simulink model "Combined_Experiment_Mar25_2020a_TorqueControl"  (R2020a)
settings: Solver=FixedStepAuto  StartTime=0.0  StopTime=tsim  FixedStep=baseRate  MaxStep=0.0001  RelTol=1e-6  AbsTol=1e-6  EnableMultiTasking=on
values from neighbouring files (symbols this model uses):
  b0 = importdata("biases_layer_0.csv")    [Run_Initializer.m]
  b1 = importdata("biases_layer_1.csv")    [Run_Initializer.m]
  b_out = importdata("biases_output.csv")    [Run_Initializer.m]
  baseRate = 0.05    [Run_Initializer.m]
  CHASER_ABSOLUTE_POSITION = true    [Run_Initializer.m]
  drop_states_ARM = [ pi/2, pi/2, 0]    [Run_Initializer.m]
  drop_states_BLACK = [ xLength/2, yLength/2, pi]    [Run_Initializer.m]
  drop_states_BLUE = [ xLength/2, yLength/2, pi]    [Run_Initializer.m]
  drop_states_RED = [ xLength/2+0.5, yLength/2, pi]    [Run_Initializer.m]
  F_Black_X_nominal = 0.2196    [Run_Initializer.m]
  F_Black_Y_nominal = 0.2825    [Run_Initializer.m]
  F_Blue_X_nominal = 0.2196    [Run_Initializer.m]
  F_Blue_Y_nominal = 0.2825    [Run_Initializer.m]
  F_red_X_nominal = 0.2196    [Run_Initializer.m]
  F_red_Y_nominal = 0.2825    [Run_Initializer.m]
  F_thrusters_BLACK = [F_Black_X_nominal; F_Black_X_nominal;                             F_Black_Y_nominal; F_Black_Y_nominal; F_Black_X_nominal;                              F_Black_X_nominal; F_Black_Y_nominal; F_Black_Y_nominal]    [Run_Initializer.m]
  F_thrusters_BLUE = [F_Blue_X_nominal; F_Blue_X_nominal;                             F_Blue_Y_nominal; F_Blue_Y_nominal; F_Blue_X_nominal;                              F_Blue_X_nominal; F_Blue_Y_nominal; F_Blue_Y_nominal]    [Run_Initializer.m]
  F_thrusters_RED = [F_red_X_nominal; F_red_X_nominal;                             F_red_Y_nominal; F_red_Y_nominal; F_red_X_nominal;                              F_red_X_nominal; F_red_Y_nominal; F_red_Y_nominal]    [Run_Initializer.m]
  Gamma1_el = 0.12    [Run_Initializer.m]
  Gamma1_sh = 0.005    [Run_Initializer.m]
  Gamma1_wr = 0.025    [Run_Initializer.m]
  Gamma2_el = 5    [Run_Initializer.m]
  Gamma2_sh = 15    [Run_Initializer.m]
  Gamma2_wr = 5    [Run_Initializer.m]
  Gamma3_el = 10    [Run_Initializer.m]
  Gamma3_sh = 40    [Run_Initializer.m]
  Gamma3_wr = 40    [Run_Initializer.m]
  Gamma4_el = 0.039    [Run_Initializer.m]
  Gamma4_sh = 0.015    [Run_Initializer.m]
  Gamma4_wr = 0.029    [Run_Initializer.m]
  Gamma5_el = 800    [Run_Initializer.m]
  Gamma5_sh = 800    [Run_Initializer.m]
  Gamma5_wr = 800    [Run_Initializer.m]
  Gamma6_el = 0.000001    (= 1e-06)    [Run_Initializer.m]
  Gamma6_sh = 0.005    [Run_Initializer.m]
  Gamma6_wr = 0.02    [Run_Initializer.m]
  HOLD_POINT_RADIUS = 0.95    [Run_Initializer.m]
  home_states_BLACK = [ xLength/2; yLength/2; 0]    [Run_Initializer.m]
  home_states_BLUE = [ xLength/2; yLength/2; 0]    [Run_Initializer.m]
  home_states_RED = [ xLength/2+0.9; yLength/2; pi]    [Run_Initializer.m]
  init_states_BLACK = [ xLength/2; yLength/2; pi]    [Run_Initializer.m]
  init_states_BLUE = [ xLength/2; yLength/2; pi]    [Run_Initializer.m]
  init_states_RED = [ xLength/2+0.9; yLength/2; pi]    [Run_Initializer.m]
  Kd_tb = 1.0    (= 1)    [Run_Initializer.m]
  Kd_tblue = 1    [Run_Initializer.m]
  Kd_tr = 1.0    (= 1)    [Run_Initializer.m]
  Kd_xb = 8    [Run_Initializer.m]
  Kd_xblue = 8    [Run_Initializer.m]
  Kd_xr = 8    [Run_Initializer.m]
  Kd_yb = 8    [Run_Initializer.m]
  Kd_yblue = 8    [Run_Initializer.m]
  Kd_yr = 8    [Run_Initializer.m]
  Kp_tb = 0.1    [Run_Initializer.m]
  Kp_tblue = 0.1    [Run_Initializer.m]
  Kp_tr = 0.1    [Run_Initializer.m]
  Kp_xb = 2    [Run_Initializer.m]
  Kp_xblue = 2    [Run_Initializer.m]
  Kp_xr = 2    [Run_Initializer.m]
  Kp_yb = 2    [Run_Initializer.m]
  Kp_yblue = 2    [Run_Initializer.m]
  Kp_yr = 2    [Run_Initializer.m]
  MAX_BODY_ANGULAR_VELOCITY = 15*180/pi    (= 859.436692696)    [Run_Initializer.m]
  MAX_VELOCITY = 0.1    [Run_Initializer.m]
  noise_variance_BLACK = 0    [Run_Initializer.m]
  noise_variance_BLUE = 0    [Run_Initializer.m]
  noise_variance_RED = 0    [Run_Initializer.m]
  Phase0_End = Phase0_Duration    (= 10)    [Run_Initializer.m]
  Phase1_End = Phase0_Duration + Phase1_Duration    (= 15)    [Run_Initializer.m]
  Phase2_End = Phase0_Duration + Phase1_Duration +                                   Phase2_Duration    (= 45)    [Run_Initializer.m]
  Phase3_End = Phase0_Duration + Phase1_Duration +                                   Phase2_Duration + Phase3_Duration    (= 560)    [Run_Initializer.m]
  Phase3_SubPhase1_End = Phase2_End + Phase3_SubPhase1_Duration    (= 105)    [Run_Initializer.m]
  Phase3_SubPhase2_End = Phase2_End + Phase3_SubPhase1_Duration +                                   Phase3_SubPhase2_Duration    (= 210)    [Run_Initializer.m]
  Phase3_SubPhase3_End = Phase2_End + Phase3_SubPhase1_Duration +                                   Phase3_SubPhase2_Duration +                                  Phase3_SubPhase3_Duration    (= 240)    [Run_Initializer.m]
  Phase3_SubPhase4_End = Phase2_End + Phase3_SubPhase1_Duration +                                   Phase3_SubPhase2_Duration +                                  Phase3_SubPhase3_Duration +                                  Phase3_SubPhase4_Duration    [Run_Initializer.m]
  Phase4_End = Phase0_Duration + Phase1_Duration +                                   Phase2_Duration + Phase3_Duration +                                   Phase4_Duration    (= 680)    [Run_Initializer.m]
  Phase5_End = Phase0_Duration + Phase1_Duration +                                   Phase2_Duration + Phase3_Duration +                                   Phase4_Duration + Phase5_Duration    (= 700)    [Run_Initializer.m]
  relevant_half_range = (upper_state_bound - lower_state_bound)/2    [Run_Initializer.m]
  relevant_state_mean = (lower_state_bound + upper_state_bound)/2    [Run_Initializer.m]
  thruster_dist2CG_BLACK = [72.80;-65.20;61.75;-79.75;65.20;-65.20;74.25;-54.75]    [Run_Initializer.m]
  thruster_dist2CG_BLUE = [83.10;-54.90;71.50;-70.00;54.90;-75.50;64.50;-64.50]    [Run_Initializer.m]
  thruster_dist2CG_RED = [69.38;-56.62;50.01;-81.49;61.12;-68.38;78.99;-52.01]    [Run_Initializer.m]
  w0 = importdata("weights_layer_0.csv")    [Run_Initializer.m]
  w1 = importdata("weights_layer_1.csv")    [Run_Initializer.m]
  w_out = importdata("weights_output.csv")    [Run_Initializer.m]
  xLength = 3.51155    [Run_Initializer.m]
  yLength = 2.41935    [Run_Initializer.m]
undefined symbols (not defined in the file or in its folder): DiscIntNeverNeededParam, model_param, platformSelection, serverRate, simMode
libraries: dspstat3 x18, raspberrypiBasiclib x9, simulink x9, dspsigops x9, embdlinuxlib x7, MainLibrary x4, mspfiltlib x3, dsparch4 x3, etargetslib x1, sensehatlib x1
(part 13 of 13)

== matlab function Combined_Experiment_Mar25_2020a_TorqueControl/Jetson Communication/Kirk Network Control (EXP)/MATLAB Function ==
  data: Pi_time input; Ax_command output; Pi_red_x input; Pi_red_y input; Pi_red_theta input; Pi_red_Vx input; Pi_red_Vy input; Pi_red_omega input; Pi_black_x input; Pi_black_y input; Pi_black_theta input; Pi_black_Vx input; Pi_black_Vy input; Pi_black_omega input; Ay_command output; Az_command output; CHASER_ABSOLUTE_POSITION parameter; relevant_state_mean parameter; relevant_half_range parameter; w0 parameter; b0 parameter; w1 parameter; b1 parameter; w_out parameter; b_out parameter; MAX_VELOCITY parameter; MAX_BODY_ANGULAR_VELOCITY parameter; ZED_Processing_Time input; ZED_Relative_X input; ZED_Relative_Y input; ZED_Yaw input; ZED_Confidence input; HOLD_POINT_RADIUS input; ZED_Relative_X_prev input; ZED_Relative_Y_prev input; ZED_Relative_Yaw_prev input
function [Ax_command, Ay_command, Az_command ] = guidance_server_sim(Pi_time, Pi_red_x, Pi_red_y, Pi_red_theta, Pi_red_Vx, Pi_red_Vy,...
                                 Pi_red_omega, Pi_black_x, Pi_black_y, Pi_black_theta, Pi_black_Vx,...
                                 Pi_black_Vy, Pi_black_omega, CHASER_ABSOLUTE_POSITION, relevant_state_mean, relevant_half_range, w0, b0, w1, b1, w_out, b_out, MAX_VELOCITY,...
                                 MAX_BODY_ANGULAR_VELOCITY, ZED_Processing_Time, ZED_Relative_X, ZED_Relative_Y, ZED_Yaw, ZED_Confidence, HOLD_POINT_RADIUS, ZED_Relative_X_prev,...
                                 ZED_Relative_Y_prev, ZED_Relative_Yaw_prev)
    
    
    Pi_red_theta = unwrap(Pi_red_theta);                         
    Pi_black_theta = unwrap(Pi_black_theta);  
    
    % Look for suddent changes in the estimate. This can be helpful for
    % cases where the ZED confidence is high but the estimate is just
    % wrong.
    
    ZED_X_Diff = abs(ZED_Relative_X-ZED_Relative_X_prev);
    ZED_Y_Diff = abs(ZED_Relative_Y-ZED_Relative_Y_prev);
    ZED_Yaw_Diff = abs(ZED_Yaw-ZED_Relative_Yaw_prev);
                             
    % Check the confidence level of the camera:
    if ZED_Confidence <= 0.8
       SPOTNet_sees_target = false;
    else
       SPOTNet_sees_target = true; 
    end
    
    % Correct the state estimates 
    
    VELOCITY_LIMIT = [MAX_VELOCITY, MAX_VELOCITY,MAX_BODY_ANGULAR_VELOCITY]; 
    
    if SPOTNet_sees_target == true
        
        
        % Calculate the inertial position of the target relative to the
        % chaser
        SPOTNet_target_x_inertial = Pi_red_x + ZED_Relative_X*cos(Pi_red_theta) - ZED_Relative_Y*sin(Pi_red_theta);
        SPOTNet_target_y_inertial = Pi_red_y + ZED_Relative_X*sin(Pi_red_theta) + ZED_Relative_Y*cos(Pi_red_theta);
        SPOTNet_target_angle_inertial = Pi_red_theta + ZED_Yaw;
        
        % Adjust the position slightly to predict the current location.
        % This would be well suited for some kind of kalman filter, where
        % we combine the simulation and vision to estimate the position.
        %SPOTNet_target_x_inertial = SPOTNet_target_x_inertial + Pi_black_Vx*ZED_Processing_Time;
        %SPOTNet_target_y_inertial = SPOTNet_target_y_inertial + Pi_black_Vy*ZED_Processing_Time;
        %SPOTNet_target_angle_inertial = SPOTNet_target_angle_inertial + Pi_black_omega*ZED_Processing_Time;
        
        relative_pose_inertial = [SPOTNet_target_x_inertial - Pi_red_x, SPOTNet_target_y_inertial - Pi_red_y, SPOTNet_target_angle_inertial - Pi_red_theta];     
        
        %Calculate desired position and velocity in the inertial frame        
        desired_position_relative_to_target_I = [-sin(SPOTNet_target_angle_inertial)*(HOLD_POINT_RADIUS), cos(SPOTNet_target_angle_inertial)*(HOLD_POINT_RADIUS), -pi/2];
        desired_position_I = [SPOTNet_target_x_inertial, SPOTNet_target_y_inertial, SPOTNet_target_angle_inertial] + desired_position_relative_to_target_I;
        desired_velocity_I = [Pi_black_Vx, Pi_black_Vy, Pi_black_omega] + cross([0,0,Pi_black_omega], desired_position_relative_to_target_I);                    
        
        % Now calculate the chaser's relative position and velocity to that desired location and velocity in the inertial frame
        chaser_position_error_inertial = desired_position_I - [Pi_red_x, Pi_red_y, Pi_red_theta];
        chaser_velocity_error_inertial = desired_velocity_I - [Pi_red_Vx, Pi_red_Vy, Pi_red_omega];                   
        policy_input = [Pi_red_x, Pi_red_y, mod(Pi_red_theta, 2*pi), Pi_red_Vx, Pi_red_Vy, Pi_red_omega, relative_pose_inertial, chaser_position_error_inertial, chaser_velocity_error_inertial];

        % Normalize the states
        normalized_policy_input = (policy_input - relevant_state_mean)./relevant_half_range;
        
        % Run the policy input through the neural network
        
        % First fully-connected layer
        layer_1 = max(0,normalized_policy_input*w0 + b0);

        % Second fully-connected layer
        layer_2 = max(0,layer_1*w1 + b1);

        % Output layer
        output = tanh(layer_2*w_out + b_out);
        
        % Convert commands
        output(1) = output(1).*0.01;
        output(2) = output(2).*0.01;
        output(3) = output(3).*0.02;
        
        % Transform back to inertial
        %output(1:2) = C_bI_red'*output(1:2)';
        
        % Cap the velocities if they exceed limits
        % Checking whether our velocity is too large AND the acceleration is trying to increase said velocity... in which case we set the desired_linear_acceleration to zero.
    	% this is in the inertial frame							   
        current_velocity = [Pi_red_Vx, Pi_red_Vy, Pi_red_omega];
        
        if abs(current_velocity(1)) > VELOCITY_LIMIT(1) && sign(output(1))==sign(current_velocity(1))
            
            output(1) = 0;
            
        end
        
        if abs(current_velocity(2)) > VELOCITY_LIMIT(2) && sign(output(2))==sign(current_velocity(2))
            
            output(2) = 0;
            
        end
        
        if abs(current_velocity(3)) > VELOCITY_LIMIT(3) && sign(output(3))==sign(current_velocity(3))
            
            output(3) = 0;
            
        end
        
    else
        
        % We don't see the target -> Use PhaseSpace only
        % Calculating the relative X and Y in the chaser's body frame using PhaseSpace
        relative_pose_inertial = [Pi_black_x - Pi_red_x, Pi_black_y - Pi_red_y, Pi_black_theta - Pi_red_theta];
        
        % Calculate the roation matrix from inertia to body
        C_bI_red = [ cos(Pi_red_theta), sin(Pi_red_theta);...
                -sin(Pi_red_theta), cos(Pi_red_theta)];
        
        % Calculate relative body pose    
        %relative_pose_body     = C_bI_red*relative_pose_inertial;
        
        % With chaser absolute position
        % policy_input = np.array([relative_pose_body[0] - self.offset_x, relative_pose_body[1] - self.offset_y, (self.SPOTNet_target_angle_inertial - Pi_red_theta - self.offset_angle)%(2*np.pi), Pi_red_x, Pi_red_y, Pi_red_theta, Pi_red_Vx, Pi_red_Vy, Pi_red_omega, Pi_black_omega])

        %############# New policy input as of Nov 9 2022                    
        % Calculate the desired X, Y, theta, Vx, Vy, omega 
        % relative to the chaser's current state
        % all in the inertial frame                 

        %Calculate desired position and velocity in the inertial frame
        desired_position_relative_to_target_I = [-sin(Pi_black_theta)*(HOLD_POINT_RADIUS), cos(Pi_black_theta)*(HOLD_POINT_RADIUS), -pi/2];
        desired_position_I = [Pi_black_x, Pi_black_y, Pi_black_theta] + desired_position_relative_to_target_I;
        desired_velocity_I = [Pi_black_Vx, Pi_black_Vy, Pi_black_omega] + cross([0,0,Pi_black_omega], desired_position_relative_to_target_I);

        % Now calculate the chaser's relative position and velocity to that desired location and velocity in the inertial frame
        chaser_position_error_inertial = desired_position_I - [Pi_red_x, Pi_red_y, Pi_red_theta];
        chaser_velocity_error_inertial = desired_velocity_I - [Pi_red_Vx, Pi_red_Vy, Pi_red_omega];
        policy_input = [Pi_red_x, Pi_red_y, mod(Pi_red_theta, 2*pi), Pi_red_Vx, Pi_red_Vy, Pi_red_omega, relative_pose_inertial, chaser_position_error_inertial, chaser_velocity_error_inertial];

        % Normalize the states
        normalized_policy_input = (policy_input - relevant_state_mean)./relevant_half_range;
        
        % Run the policy input through the neural network
        
        % First fully-connected layer
        layer_1 = max(0,normalized_policy_input*w0 + b0);

        % Second fully-connected layer
        layer_2 = max(0,layer_1*w1 + b1);

        % Output layer
        output = tanh(layer_2*w_out + b_out);
        
        % Convert commands
        output(1) = output(1).*0.01;
        output(2) = output(2).*0.01;
        output(3) = output(3).*0.02;
        
        % Transform back to inertial
        output(1:2) = C_bI_red'*output(1:2)';
        
        % Cap the velocities if they exceed limits
        % Checking whether our velocity is too large AND the acceleration is trying to increase said velocity... in which case we set the desired_linear_acceleration to zero.
    	% this is in the inertial frame							   
        current_velocity = [Pi_red_Vx, Pi_red_Vy, Pi_red_omega];
        
        if abs(current_velocity(1)) > VELOCITY_LIMIT(1) && sign(output(1))==sign(current_velocity(1))
            
            output(1) = 0;
            
        end
        
        if abs(current_velocity(2)) > VELOCITY_LIMIT(2) && sign(output(2))==sign(current_velocity(2))
            
            output(2) = 0;
            
        end
        
        if abs(current_velocity(3)) > VELOCITY_LIMIT(3) && sign(output(3))==sign(current_velocity(3))
            
            output(3) = 0;
            
        end
        
    end
    
    Ax_command = output(1);
    Ay_command = output(2);
    Az_command = output(3);
                             
end

== matlab function Combined_Experiment_Mar25_2020a_TorqueControl/From Force//Torque to PWM Signal/Change BLUE Behavior/Calculate Thruster ON//OFF/MATLAB Function ==
  data: H output; thruster_dist2CG_BLUE parameter; F_thrusters_BLUE parameter
function H = MakeH(thruster_dist2CG_BLUE,F_thrusters_BLUE)

Vec1 = [ -1
         -1
          0 
          0
          1
          1
          0
          0 ];
      
Vec2 = [  0
          0
          1
          1
          0
          0
         -1
         -1 ];
     
Vec3 = thruster_dist2CG_BLUE./1000;

Mat1 = [Vec1, Vec2, Vec3]';

Mat2 = diag((F_thrusters_BLUE./2));

H    = Mat1*Mat2;

end

== matlab function Combined_Experiment_Mar25_2020a_TorqueControl/Phase #3: Experiment/Change RED Behavior/Sub-Phase #4/RED+ARM/Transpose Jacobian Controller/Arm Controller/MATLAB Function1 ==
  data: qe3 input; qe3i input; qe3d input; tau3_aux output
function tau3_aux  = fcn(qe3, qe3i, qe3d)
%#codegen

% Calculate the required angle for the joint plane to be parallel with the
% dock

% Multiply by some gains to get a torque
tau3_aux = qe3*75 + qe3i*20 + qe3d*10;

end

== matlab function Combined_Experiment_Mar25_2020a_TorqueControl/Phase #3: Experiment/Change RED Behavior/Sub-Phase #4/RED+ARM/MATLAB Function1 ==
  data: Sim_Time input; Control_Mode output
function Control_Mode = SwitchModes(Sim_Time)

    if Sim_Time < 2
        
        Control_Mode = 0;
        
    else 
        
        Control_Mode = 2;
        
    end

end

== matlab function Combined_Experiment_Mar25_2020a_TorqueControl/Phase #4: Return Home/Change RED Behavior/RED+ARM/MATLAB Function1 ==
  data: Sim_Time input; Control_Mode output
function Control_Mode = SwitchModes(Sim_Time)

    if Sim_Time < 2
        
        Control_Mode = 0;
        
    else 
        
        Control_Mode = 1;
        
    end

end

== matlab function Combined_Experiment_Mar25_2020a_TorqueControl/Simulate Plant Dynamics/RED and ARM Dynamics/RED + ARM/RED + ARM Dynamics/MATLAB Function ==
  data: Control_Mode input; Shoulder_Torque output; Shoulder_Command input; Elbow_Command input; Wrist_Command input; Elbow_Torque output; Wrist_Torque output; Shoulder_Angle input; Elbow_Angle input; Wrist_Angle input
function [Shoulder_Torque, Elbow_Torque, Wrist_Torque] = Check_Inputs(Control_Mode, Shoulder_Command, Elbow_Command, Wrist_Command,...
                                                               Shoulder_Angle, Elbow_Angle, Wrist_Angle)

    

    if Control_Mode == 2
        
        Shoulder_Torque = Shoulder_Command;
        Elbow_Torque = Elbow_Command;
        Wrist_Torque = Wrist_Command;
        
    else
        
        Shoulder_Torque = 0;
        Elbow_Torque = 0;
        Wrist_Torque = 0;
        
    end
        

end

== matlab function Combined_Experiment_Mar25_2020a_TorqueControl/Phase #3: Experiment/Change RED Behavior/Sub-Phase #4/Hough Control/MATLAB Function2 ==
  data: Oy output; z input; Ox output
function [Oy, Ox]   = C3( z )
%C3 gives the rotation matrix about the z-axis for an angle 'z'
%   z - the angle about the z-axis which you rotate
%   A - the rotation matrix

Ox = [cos(z) sin(z); -sin(z) cos(z)]*[1;0];
Oy = [cos(z) sin(z); -sin(z) cos(z)]*[0;1];
end

== matlab function Combined_Experiment_Mar25_2020a_TorqueControl/Phase #3: Experiment/Change RED Behavior/Sub-Phase #4/RED+ARM/Transpose Jacobian Controller/End-Effector Position ==
  data: y output; q input
function y = ForwardKinematics(q)
%#codegen

phi= 73.2749*pi/180;          % ARM Phi
b0= 0.25;                     % ARM b0
a1= 0.196822;                 % ARM a1
b1= 0.107678;                 % ARM b1
a2= 0.198152;                 % ARM a2
b2= 0.106348;                 % ARM b2
a3= 0.062097;                 % ARM a3
b3= 0.025153;                 % ARM b3

l1     = a1+b1;
l2     = a2+b2;
l3     = a3+b3;

% Define Variables
q1 = q(1);
q2 = q(2);
q3 = q(3);

% Calculate End-Effector Position & Velocity
y = [ (b0)*cos(phi) + (l1)*cos(pi/2+q1) + (l2)*cos(pi/2+q1+q2) + (l3)*cos(pi/2+q1+q2+q3),...
      (b0)*sin(phi) + (l1)*sin(pi/2+q1) + (l2)*sin(pi/2+q1+q2) + (l3)*sin(pi/2+q1+q2+q3)];
  
end

== matlab function Combined_Experiment_Mar25_2020a_TorqueControl/From Force//Torque to PWM Signal/Change BLUE Behavior/Calculate Thruster ON//OFF/MATLAB Function1 ==
  data: H output; thruster_dist2CG_BLUE parameter; F_thrusters_BLUE parameter
function H = MakeH(thruster_dist2CG_BLUE,F_thrusters_BLUE)

Vec1 = [ -1
         -1
          0 
          0
          1
          1
          0
          0 ];
      
Vec2 = [  0
          0
          1
          1
          0
          0
         -1
         -1 ];
     
Vec3 = thruster_dist2CG_BLUE./1000;

Mat1 = [Vec1, Vec2, Vec3]';

Mat2 = diag((F_thrusters_BLUE./2));

H    = Mat1*Mat2;

end

== matlab function Combined_Experiment_Mar25_2020a_TorqueControl/Phase #3: Experiment/Change RED Behavior/Sub-Phase #4/RED+ARM/Transpose Jacobian Controller/Error Signal/End-Effector Position1 ==
  data: y output; q input; u input
function y = ForwardKinematics(q, u)
%#codegen
theta = q(3);

C_bI_RED = [  cos(theta) sin(theta)
            -sin(theta) cos(theta) ];
                                 
y  = C_bI_RED*u;  
end

== matlab function Combined_Experiment_Mar25_2020a_TorqueControl/Phase #3: Experiment/Change RED Behavior/Sub-Phase #4/RED+ARM/Transpose Jacobian Controller/Transpose Generalized Jacobian /Inertia Function  ==
  data: InertiaS output; x input
function InertiaS = InertiaFunc3LINK(x)
%INERTIAFUNC3LINK
%    INERTIAS = INERTIAFUNC3LINK(I0,I1,I2,I3,A1,A2,A3,B0,B1,B2,M0,M1,M2,M3,PHI,Q0,Q1,Q2,Q3)

%    This function was generated by the Symbolic Math Toolbox version 8.5.
%    15-Mar-2022 15:58:51

q0 = 0;
q1 = x(1);
q2 = x(2);
q3 = x(3);

m0            = 13.0720;     % RED Mass
I0            = 0.2405;      % RED Inertia
phi           = 73.2749*180/pi; % ARM Phi
b0            = 0.25;        % ARM b0
a1            = 0.196822;    % ARM a1
b1            = 0.107678;    % ARM b1
a2            = 0.198152;    % ARM a2
b2            = 0.106348;    % ARM b2
a3            = 0.062097;    % ARM a3
b3            = 0.025153;    % ARM b3
m1            = 0.345;       % ARM m1
m2            = 0.335;       % ARM m2
m3            = 0.111;       % ARM m3
I1            = 0.003704;    % ARM I1
I2            = 0.003506;    % ARM I2
I3            = 0.000106;    % ARM I3

t2 = cos(q2);
t3 = cos(q3);
t4 = a1+b1;
t5 = a2+b2;
t6 = a1.*m1;
t7 = a2.*m2;
t8 = a2.*m3;
t9 = a3.*m3;
t10 = b0.*m1;
t11 = b0.*m2;
t12 = b0.*m3;
t13 = b2.*m3;
t14 = phi+q0;
t15 = q0+q1;
t16 = q2+q3;
t17 = a1.^2;
t18 = a2.^2;
t19 = a3.^2;
t20 = b0.^2;
t21 = b1.^2;
t22 = b2.^2;
t48 = -phi;
t49 = -q1;
t50 = m0+m1+m2+m3;
t76 = a1.*b1.*m2.*2.0;
t77 = a1.*b1.*m3.*2.0;
t23 = a1.*t7;
t24 = a1.*t8;
t25 = a1.*t9;
t26 = a3.*t8;
t27 = b0.*t6;
t28 = a1.*t11;
t29 = a1.*t12;
t30 = b0.*t7;
t31 = b0.*t8;
t32 = b1.*t7;
t33 = a1.*t13;
t34 = b1.*t8;
t35 = b0.*t9;
t36 = b1.*t9;
t37 = b2.*t9;
t38 = b1.*t11;
t39 = b1.*t12;
t40 = b2.*t12;
t41 = b1.*t13;
t42 = cos(t14);
t43 = cos(t15);
t44 = cos(t16);
t45 = q2+t15;
t46 = sin(t14);
t47 = sin(t15);
t52 = t15+t16;
t54 = -t6;
t55 = -t7;
t56 = -t8;
t57 = -t9;
t58 = -t10;
t59 = -t11;
t60 = -t12;
t61 = -t13;
t62 = a1.*t6;
t63 = m2.*t17;
t64 = m3.*t17;
t65 = a2.*t7;
t66 = a2.*t8;
t67 = a3.*t9;
t69 = m2.*t21;
t70 = m3.*t21;
t71 = b2.*t13;
t81 = b2.*t8.*2.0;
t85 = m2.*t4;
t86 = m3.*t4;
t87 = m3.*t5;
t94 = phi+t49;
t95 = q1+q2+t48;
t101 = q1+t16+t48;
t106 = t10+t11+t12;
t51 = cos(t45);
t53 = sin(t45);
t68 = t67;
t72 = t23.*2.0;
t73 = t24.*2.0;
t74 = t25.*2.0;
t75 = t26.*2.0;
t78 = t32.*2.0;
t79 = t33.*2.0;
t80 = t34.*2.0;
t82 = t36.*2.0;
t83 = t37.*2.0;
t84 = t41.*2.0;
t88 = cos(t52);
t89 = -t30;
t90 = -t31;
t91 = -t35;
t92 = -t40;
t93 = sin(t52);
t96 = sin(t94);
t98 = -t85;
t99 = -t86;
t100 = -t87;
t102 = sin(t95);
t103 = t25+t36;
t104 = t26+t37;
t105 = sin(t101);
t115 = t42.*t106;
t118 = t55+t56+t61;
t119 = t58+t59+t60;
t125 = t27+t28+t29+t38+t39;
t126 = -t46.*t106;
t129 = -t43.*(t6+t85+t86);
t130 = -t47.*(t6+t85+t86);
t131 = t23+t24+t32+t33+t34+t41;
t97 = I3+t68;
t107 = t74+t82;
t108 = t75+t83;
t109 = t57.*t88;
t110 = t57.*t93;
t111 = t3.*t104;
t112 = t55+t100;
t113 = t44.*t103;
t117 = t91.*t105;
t120 = -t53.*(t7+t87);
t121 = t89+t90+t92;
t122 = -t51.*(t7+t87);
t124 = t54+t98+t99;
t127 = -t51.*(t7+t8+t13);
t128 = -t53.*(t7+t8+t13);
t133 = t2.*t131;
t134 = -t102.*(t30+t31+t40);
t135 = t96.*t125;
t136 = t72+t73+t78+t79+t80+t84;
t114 = t3.*t108;
t116 = t44.*t107;
t123 = t97+t111;
t132 = I2+t65+t66+t71+t81+t97;
t138 = t2.*t136;
t139 = t109+t127;
t140 = t110+t128;
t142 = t110+t120+t130;
t143 = t109+t122+t129;
t137 = t113+t123;
t144 = I1+t62+t63+t64+t69+t70+t76+t77+t132;
t145 = t115+t142;
t146 = t126+t143;
t147 = t113+t114+t132+t133;
t141 = t117+t137;
t148 = t117+t134+t147;
t149 = t114+t116+t117+t134+t135+t138+t144;
InertiaS = reshape([t50,0.0,t146,t143,t139,t109,0.0,t50,t145,t142,t140,t110,t146,t145,I0+t114+t116+t135.*2.0+t138+t144+b0.*t10+b0.*t11+b0.*t12-t35.*t105.*2.0-t102.*(t30.*2.0+t31.*2.0+t40.*2.0),t149,t148,t141,t143,t142,t149,t114+t116+t138+t144,t147,t137,t139,t140,t148,t147,t114+t132,t123,t109,t110,t141,t137,t123,t97],[6,6]);

end

== matlab function Combined_Experiment_Mar25_2020a_TorqueControl/Phase #3: Experiment/Change RED Behavior/Sub-Phase #4/Hough Control/MATLAB Function3 ==
  data: z input; Ox output
function Ox    = C3( z )
%C3 gives the rotation matrix about the z-axis for an angle 'z'
%   z - the angle about the z-axis which you rotate
%   A - the rotation matrix

Ox = [cos(z) sin(z); -sin(z) cos(z)]*[1;0];
end

== matlab function Combined_Experiment_Mar25_2020a_TorqueControl/Phase #3: Experiment/Change RED Behavior/Sub-Phase #4/Hough Control/MATLAB Function4 ==
  data: Oy input; e_out output; e_in input
function e_out = fcn(Oy, e_in)

a = sign(Oy'*e_in);
e_out = -a*norm(e_in);

== matlab function Combined_Experiment_Mar25_2020a_TorqueControl/Phase #3: Experiment/Change RED Behavior/Sub-Phase #3 /Hough Control/MATLAB Function3 ==
  data: z input; Ox output
function Ox    = C3( z )
%C3 gives the rotation matrix about the z-axis for an angle 'z'
%   z - the angle about the z-axis which you rotate
%   A - the rotation matrix

Ox = [cos(z) sin(z); -sin(z) cos(z)]*[1;0];
end

== matlab function Combined_Experiment_Mar25_2020a_TorqueControl/Phase #3: Experiment/Change RED Behavior/Sub-Phase #3 /Hough Control/MATLAB Function4 ==
  data: Oy input; e_out output; e_in input
function e_out = fcn(Oy, e_in)

a = sign(Oy'*e_in);
e_out = -a*norm(e_in);

== matlab function Combined_Experiment_Mar25_2020a_TorqueControl/Phase #3: Experiment/Change RED Behavior/Sub-Phase #3 /calculate_mass_matrix ==
  data: M output
function M  = generate_M()
  
    m0                 = 13.80;     % RED Mass
    I0                = 0.242150;      % RED Inertia;
   


    M = [m0 0 0
         0 m0 0
         0 0 I0];

end
% Artificially setting M_31 and M_32 to zero, such that the feedforward
% controller does not think a torque needs to be applied to the base to
% counteract the torque needed to maintain the angular acceleration of the
% links when the base has a linear acceleration. No torque is applied to keep the links at their linear
% acceleration because friction does this for us.

% The original matrix
% M = reshape([t17,0.0,t30,-t86-t87-t88,-t88-t13.*t28,-t88,...
%     0.0,t17,t33,-t89-t90-t91,-t91-t24.*t28,-t91,...
%     t30,t33,...
%     I0+I1+I2+I3+t46+t51+t57+t64+t65+t66+t67+t68+t70+t71+t72+t74+t75+t76+t77+t59.*(a1.*b0.*m1.*2.0+a1.*b0.*m2.*2.0+a1.*b0.*m3.*2.0+b0.*b1.*m2.*2.0+b0.*b1.*m3.*2.0)+m1.*t36+m2.*t36+m3.*t36-t61.*(a2.*b0.*m2.*2.0+a2.*b0.*m3.*2.0+b0.*b2.*m3.*2.0)-a3.*b0.*m3.*t63.*2.0,t99,I2+I3+t51+t67+t68+t70+t74+t77+t85+t107-t112-t113,I3+t70+t85+t111-t113,-t7.*t8-t13.*t14-a3.*m3.*t16,    -t8.*t23-t14.*t24-a3.*m3.*t25,t99,I1+I2+I3+t46+t51+t57+t64+t65+t66+t67+t68+t70+t71+t72+t74+t75+t76+t77,t114,t115,-t13.*t28-a3.*m3.*t16,-t24.*t28-a3.*m3.*t25,I2+I3+t51+t67+t68+t70+t74+t77+t85+t107-t61.*t81-a3.*b0.*m3.*t63,t114,I2+I3+t51+t67+t68+t70+t74+t77,t116,-a3.*m3.*t16,-a3.*m3.*t25,I3+t70+t85+t111-a3.*b0.*m3.*t63,t115,t116,I3+t70],[6,6]);

== matlab function Combined_Experiment_Mar25_2020a_TorqueControl/Phase #3: Experiment/Change RED Behavior/Sub-Phase #2 /Hough Control/MATLAB Function3 ==
  data: z input; Ox output
function Ox    = C3( z )
%C3 gives the rotation matrix about the z-axis for an angle 'z'
%   z - the angle about the z-axis which you rotate
%   A - the rotation matrix

Ox = [cos(z) sin(z); -sin(z) cos(z)]*[1;0];
end

== matlab function Combined_Experiment_Mar25_2020a_TorqueControl/Phase #3: Experiment/Change RED Behavior/Sub-Phase #4/RED+ARM/Transpose Jacobian Controller/Transpose Generalized Jacobian /MATLAB Function ==
  data: q input; J output; InertiaS input
function J  = fcn(q, InertiaS)
%#codegen

% Source: http://ieeexplore.ieee.org.proxy.library.carleton.ca/stamp/stamp.jsp?tp=&arnumber=34766
q0 = 0;
q1     = q(1);
q2     = q(2);
q3     = q(3);

m0            = 13.0720;     % RED Mass
I0            = 0.2405;      % RED Inertia
phi           = 73.2749*180/pi; % ARM Phi
b0            = 0.25;        % ARM b0
a1            = 0.196822;    % ARM a1
b1            = 0.107678;    % ARM b1
a2            = 0.198152;    % ARM a2
b2            = 0.106348;    % ARM b2
a3            = 0.062097;    % ARM a3
b3            = 0.025153;    % ARM b3
m1            = 0.345;       % ARM m1
m2            = 0.335;       % ARM m2
m3            = 0.111;       % ARM m3
I1            = 0.003704;    % ARM I1
I2            = 0.003506;    % ARM I2
I3            = 0.000106;    % ARM I3
l1     = a1+b1;
l2     = a2+b2;
l3     = a3+b3;

w = m0+m1+m2+m3;

% J = [ 1, 0, - l3*sin(q0 + q1 + q2 + q3) - b0*sin(phi + q0) - l1*sin(q0 + q1) - l2*sin(q0 + q1 + q2), - l3*sin(q0 + q1 + q2 + q3) - l1*sin(q0 + q1) - l2*sin(q0 + q1 + q2), - l3*sin(q0 + q1 + q2 + q3) - l2*sin(q0 + q1 + q2), -l3*sin(q0 + q1 + q2 + q3)
%       0, 1,   l3*cos(q0 + q1 + q2 + q3) + b0*cos(phi + q0) + l1*cos(q0 + q1) + l2*cos(q0 + q1 + q2),   l3*cos(q0 + q1 + q2 + q3) + l1*cos(q0 + q1) + l2*cos(q0 + q1 + q2),   l3*cos(q0 + q1 + q2 + q3) + l2*cos(q0 + q1 + q2),  l3*cos(q0 + q1 + q2 + q3)];

% Contants
K0     = m0*b0/w;
K1     = (m0*l1 + m1*b1)/w;
K2     = ((m0+m1)*l2 + m2*b2)/w;
K3     = ((m0+m1+m2)*l3 + m3*b3)/w;

% Trigonometric simplifications
s0     = sin(phi);
s1     = sin(pi/2+q1);
s2     = sin(pi/2+q1+q2);
s3     = sin(pi/2+q1+q2+q3);
c0     = cos(phi);
c1     = cos(pi/2+q1);
c2     = cos(pi/2+q1+q2);
c3     = cos(pi/2+q1+q2+q3);

% Jacobian for the base (specific)       
Jm     = [ -K1*s1-K2*s2-K3*s3 -K2*s2-K3*s3 -K3*s3 
            K1*c1+K2*c2+K3*c3  K2*c2+K3*c3  K3*c3  ];

% Jacobian for the manipulator (specific)
Js     = [ -K0*b0*s0-K1*l1*s1-K2*l2*s2-K3*l3*s3
            K0*b0*c0+K1*l1*c1+K2*l2*c2+K3*l3*c3 ];

% More constants
H      = InertiaS;
                      
Is     = H(3,3);
Im     = [H(3,4), H(3,5), H(3,6)];

% Calculate generalized Jacobian
J      = Jm - Js*(Is\Im);  

end

== matlab function Combined_Experiment_Mar25_2020a_TorqueControl/Phase #3: Experiment/Change RED Behavior/Sub-Phase #4/RED+ARM/MATLAB Function ==
  data: RED input; p_red_target output; BLACK input
function p_red_target = fcn(RED, BLACK)

    Pi_red_x = RED(1);
    Pi_red_y = RED(2);
    Pi_red_theta = RED(3);
    Pi_black_x = BLACK(1);
    Pi_black_y = BLACK(2);
    Pi_black_theta = BLACK(3); 
    
    % Define the rotation matrices for the first and second satellites
    R_red = [cos(Pi_red_theta) -sin(Pi_red_theta) 0; sin(Pi_red_theta) cos(Pi_red_theta) 0; 0 0 1];
    R_black = [cos(Pi_black_theta) -sin(Pi_black_theta) 0; sin(Pi_black_theta) cos(Pi_black_theta) 0; 0 0 1];

    % Define the offset vector for the target location
    v_target_body = [0.0743; 0.2288; 0];

    % Rotate the offset vector into the inertial frame
    v_target_inertial = R_black * v_target_body;

    % Compute the position of the center of mass of the second satellite in the inertial frame
    p_black_inertial = [Pi_black_x; Pi_black_y; 0] + v_target_inertial;

    % Compute the position of the center of mass of the second satellite in the first satellite's frame
    p_black_relative = R_red' * (p_black_inertial - [Pi_red_x; Pi_red_y; 0]);

    % Compute the position of the target in the first satellite's frame
    p_red_target = p_black_relative;
    
    % Add a bit to the x-direction for more oumph
    p_red_target(1) = p_red_target(1) + 0.07;
    p_red_target(2) = p_red_target(2) - 0.08;
   
end

== matlab function Combined_Experiment_Mar25_2020a_TorqueControl/Phase #3: Experiment/Change RED Behavior/Sub-Phase #2 /Hough Control/MATLAB Function4 ==
  data: Oy input; e_out output; e_in input
function e_out = fcn(Oy, e_in)

a = sign(Oy'*e_in);
e_out = -a*norm(e_in);

== matlab function Combined_Experiment_Mar25_2020a_TorqueControl/From Force//Torque to PWM Signal/Change BLUE Behavior/Calculate Thruster ON//OFF/MATLAB Function2 ==
  data: ThrustPer_Final output; ThrustPer input
function ThrustPer_Final  = ThrusterSat(ThrustPer)

ValveTime       = 0.007;
TControl        = 0.1;
ThrustPer_Final = zeros(8,1);

if max(ThrustPer) > 1
    ThrustPer_Sat = ThrustPer/max(ThrustPer);
else
    ThrustPer_Sat = ThrustPer;
end

for i = 1:8
    if ThrustPer_Sat(i) > ValveTime/TControl 
        ThrustPer_Final(i) = ThrustPer_Sat(i);
    else
        ThrustPer_Final(i) = 0;
    end
end
   

end

== matlab function Combined_Experiment_Mar25_2020a_TorqueControl/Phase #3: Experiment/Change RED Behavior/Sub-Phase #2 /calculate_mass_matrix ==
  data: M output
function M  = generate_M()
  
    m0                 = 13.80;     % RED Mass
    I0                = 0.242150;      % RED Inertia;
   


    M = [m0 0 0
         0 m0 0
         0 0 I0];

end
% Artificially setting M_31 and M_32 to zero, such that the feedforward
% controller does not think a torque needs to be applied to the base to
% counteract the torque needed to maintain the angular acceleration of the
% links when the base has a linear acceleration. No torque is applied to keep the links at their linear
% acceleration because friction does this for us.

% The original matrix
% M = reshape([t17,0.0,t30,-t86-t87-t88,-t88-t13.*t28,-t88,...
%     0.0,t17,t33,-t89-t90-t91,-t91-t24.*t28,-t91,...
%     t30,t33,...
%     I0+I1+I2+I3+t46+t51+t57+t64+t65+t66+t67+t68+t70+t71+t72+t74+t75+t76+t77+t59.*(a1.*b0.*m1.*2.0+a1.*b0.*m2.*2.0+a1.*b0.*m3.*2.0+b0.*b1.*m2.*2.0+b0.*b1.*m3.*2.0)+m1.*t36+m2.*t36+m3.*t36-t61.*(a2.*b0.*m2.*2.0+a2.*b0.*m3.*2.0+b0.*b2.*m3.*2.0)-a3.*b0.*m3.*t63.*2.0,t99,I2+I3+t51+t67+t68+t70+t74+t77+t85+t107-t112-t113,I3+t70+t85+t111-t113,-t7.*t8-t13.*t14-a3.*m3.*t16,    -t8.*t23-t14.*t24-a3.*m3.*t25,t99,I1+I2+I3+t46+t51+t57+t64+t65+t66+t67+t68+t70+t71+t72+t74+t75+t76+t77,t114,t115,-t13.*t28-a3.*m3.*t16,-t24.*t28-a3.*m3.*t25,I2+I3+t51+t67+t68+t70+t74+t77+t85+t107-t61.*t81-a3.*b0.*m3.*t63,t114,I2+I3+t51+t67+t68+t70+t74+t77,t116,-a3.*m3.*t16,-a3.*m3.*t25,I3+t70+t85+t111-a3.*b0.*m3.*t63,t115,t116,I3+t70],[6,6]);

== matlab function Combined_Experiment_Mar25_2020a_TorqueControl/Phase #3: Experiment/Change RED Behavior/Sub-Phase #1/Hough Control/MATLAB Function3 ==
  data: z input; Ox output
function Ox    = C3( z )
%C3 gives the rotation matrix about the z-axis for an angle 'z'
%   z - the angle about the z-axis which you rotate
%   A - the rotation matrix

Ox = [cos(z) sin(z); -sin(z) cos(z)]*[1;0];
end

== matlab function Combined_Experiment_Mar25_2020a_TorqueControl/Phase #3: Experiment/Change BLACK Behavior/Sub-Phase #1/Hough Control/MATLAB Function4 ==
  data: Oy input; e_out output; e_in input
function e_out = fcn(Oy, e_in)

a = sign(Oy'*e_in);
e_out = -a*norm(e_in);

== matlab function Combined_Experiment_Mar25_2020a_TorqueControl/Phase #3: Experiment/Change RED Behavior/Sub-Phase #1/Hough Control/MATLAB Function4 ==
  data: Oy input; e_out output; e_in input
function e_out = fcn(Oy, e_in)

a = sign(Oy'*e_in);
e_out = -a*norm(e_in);

== matlab function Combined_Experiment_Mar25_2020a_TorqueControl/Phase #3: Experiment/Change RED Behavior/Sub-Phase #1/calculate_mass_matrix ==
  data: M output
function M  = generate_M()
  
    m0                 = 13.80;     % RED Mass
    I0                = 0.242150;      % RED Inertia;
   


    M = [m0 0 0
         0 m0 0
         0 0 I0];

end
% Artificially setting M_31 and M_32 to zero, such that the feedforward
% controller does not think a torque needs to be applied to the base to
% counteract the torque needed to maintain the angular acceleration of the
% links when the base has a linear acceleration. No torque is applied to keep the links at their linear
% acceleration because friction does this for us.

% The original matrix
% M = reshape([t17,0.0,t30,-t86-t87-t88,-t88-t13.*t28,-t88,...
%     0.0,t17,t33,-t89-t90-t91,-t91-t24.*t28,-t91,...
%     t30,t33,...
%     I0+I1+I2+I3+t46+t51+t57+t64+t65+t66+t67+t68+t70+t71+t72+t74+t75+t76+t77+t59.*(a1.*b0.*m1.*2.0+a1.*b0.*m2.*2.0+a1.*b0.*m3.*2.0+b0.*b1.*m2.*2.0+b0.*b1.*m3.*2.0)+m1.*t36+m2.*t36+m3.*t36-t61.*(a2.*b0.*m2.*2.0+a2.*b0.*m3.*2.0+b0.*b2.*m3.*2.0)-a3.*b0.*m3.*t63.*2.0,t99,I2+I3+t51+t67+t68+t70+t74+t77+t85+t107-t112-t113,I3+t70+t85+t111-t113,-t7.*t8-t13.*t14-a3.*m3.*t16,    -t8.*t23-t14.*t24-a3.*m3.*t25,t99,I1+I2+I3+t46+t51+t57+t64+t65+t66+t67+t68+t70+t71+t72+t74+t75+t76+t77,t114,t115,-t13.*t28-a3.*m3.*t16,-t24.*t28-a3.*m3.*t25,I2+I3+t51+t67+t68+t70+t74+t77+t85+t107-t61.*t81-a3.*b0.*m3.*t63,t114,I2+I3+t51+t67+t68+t70+t74+t77,t116,-a3.*m3.*t16,-a3.*m3.*t25,I3+t70+t85+t111-a3.*b0.*m3.*t63,t115,t116,I3+t70],[6,6]);

== matlab function Combined_Experiment_Mar25_2020a_TorqueControl/From Force//Torque to PWM Signal/Change BLUE Behavior/Calculate Thruster ON//OFF/MATLAB Function6 ==
  data: thrust_decay_factor output; PWMs input; thruster_count_threshold parameter; count output
function [thrust_decay_factor, count]  = check_thrust_decay(PWMs,thruster_count_threshold)

% normalize PWMs
if max(PWMs) > 1
    PWMs = PWMs/max(PWMs);
end

count = sum(PWMs > thruster_count_threshold);

positives_only = max(PWMs,0);
sum_of_duty_cycles = sum(positives_only);

average_duty_cycle_per_thruster = sum_of_duty_cycles/count;

% Look up the thrust decay for this average duty cycle
if (average_duty_cycle_per_thruster < 0.3) || (count == 0)
    thrust_decay_factor = 1;
else
    thrust_decay_factor = max(0.6 - 2*average_duty_cycle_per_thruster + 1, 0.5);   
end
